simulink model "Robot_arm_position_control"  (Simulink 7.6)
settings: Solver=ode45  StartTime=0.0  StopTime=100  RelTol=1e-3
libraries: simulink x6, dspmtrx3 x1, powerlib x1
settings Model: Creator=Green  LastModifiedBy=Green

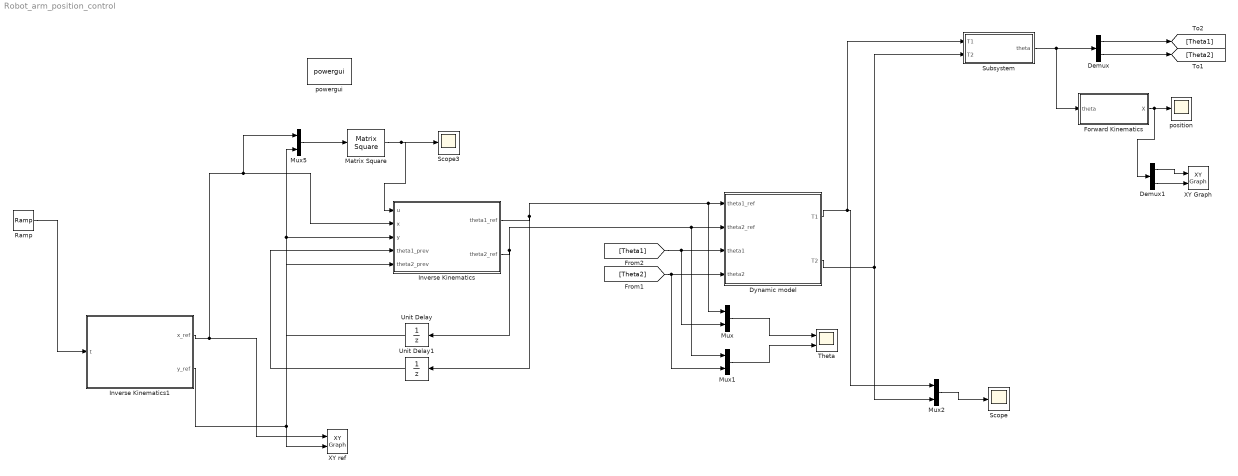
== system Robot_arm_position_control ==
  Demux : Demux  Outputs=2
  Demux1 : Demux  Outputs=2
  Dynamic model : Subsystem
  Forward Kinematics : Subsystem
  Inverse Kinematics : Stateflow chart  TreatAsAtomicUnit=on
  Inverse Kinematics1 : Stateflow chart  TreatAsAtomicUnit=on
  Matrix Square : dspmtrx3/Matrix Square  SystemSampleTime=-1  OutMin=[]  OutMax=[]
  Mux{,1..2,5} (4 alike) : Mux  Inputs=2
  Ramp : simulink/Sources/Ramp  SystemSampleTime=-1  slope=0.1  start=0  X0=0
  Scope : Scope
      settings: YMin=-1.1e+018  YMax=1.1e+018  SaveName=ScopeData2
  Scope3 : Scope
      settings: YMin=0.13  YMax=0.13  SaveName=ScopeData11
  Subsystem : Subsystem
  Theta : Scope  NumInputPorts=2
      settings: YMin=0.5~-1.2  YMax=1.45~0.7  SaveName=theta_graph  DataFormat=Structure
  Unit Delay : UnitDelay  SampleTime=-1
  Unit Delay1 : UnitDelay  SampleTime=-1
  XY Graph : simulink/Sinks/XY Graph  SystemSampleTime=-1  xmin=-0.5  xmax=0.5  ymin=-0.5  ymax=0.5  st=-1
  XY ref : simulink/Sinks/XY Graph  SystemSampleTime=-1  xmin=-0.5  xmax=0.5  ymin=-0.5  ymax=0.5  st=-1
  position : Scope
      settings: YMin=-0.05  YMax=0.4  SaveName=XY_graph  DataFormat=Array
  powergui : powerlib/powergui  Priority=1  SystemSampleTime=-1  SimulationMode=Discrete  SampleTime=50e-8  frequency=60  SPID=off  DisableSnubberDevices=off  DisableRonSwitches=off  DisableVfSwitches=off  SwTol=0  Interpol=off  frequencyindice=60  echomessages=off  HookPort=off  DisplayEquations=off  FunctionMessages=off  EnableUseOfTLC=off  x0status=blocks  RestoreLinks=warning  ResistiveCurrentMeasurement=off  Ylog=off  Xlog=on  ShowGrid=off  save=off  variable=ZData  ZoomFFT=off  StartTime=0.0  cycles=1  DisplayStyle=1  FreqAxis=off  MaxFrequency=1000  frequencyindicesteady=1  display=off  methode=off
  wires:
  Dynamic model/1(T1) -> Subsystem/1(T1), Mux2/1
  Dynamic model/2(T2) -> Subsystem/2(T2), Mux2/2
  [Theta2] -> Dynamic model/4(theta2), Mux1/2
  [Theta1] -> Dynamic model/3(theta1), Mux/2
  Inverse Kinematics/2(theta2_ref) -> Dynamic model/2(theta2_ref), Mux1/1, Unit Delay/1
  Mux/1 -> Theta/1
  Mux1/1 -> Theta/2
  Subsystem/1(theta) -> Demux/1, Forward Kinematics/1(theta)
  Demux/1 -> [Theta1]
  Demux/2 -> [Theta2]
  Mux2/1 -> Scope/1
  Inverse Kinematics/1(theta1_ref) -> Unit Delay1/1, Dynamic model/1(theta1_ref), Mux/1
  Unit Delay1/1 -> Inverse Kinematics/4(theta1_prev)
  Forward Kinematics/1(X) -> position/1, Demux1/1
  Demux1/1 -> XY Graph/1
  Demux1/2 -> XY Graph/2
  Mux5/1 -> Matrix Square/1
  Matrix Square/1 -> Scope3/1, Inverse Kinematics/1(u)
  Unit Delay/1 -> Inverse Kinematics/5(theta2_prev)
  Ramp/1 -> Inverse Kinematics1/1(t)
  Inverse Kinematics1/1(x_ref) -> XY ref/1, Inverse Kinematics/2(x), Mux5/1
  Inverse Kinematics1/2(y_ref) -> XY ref/2, Mux5/2, Inverse Kinematics/3(y)

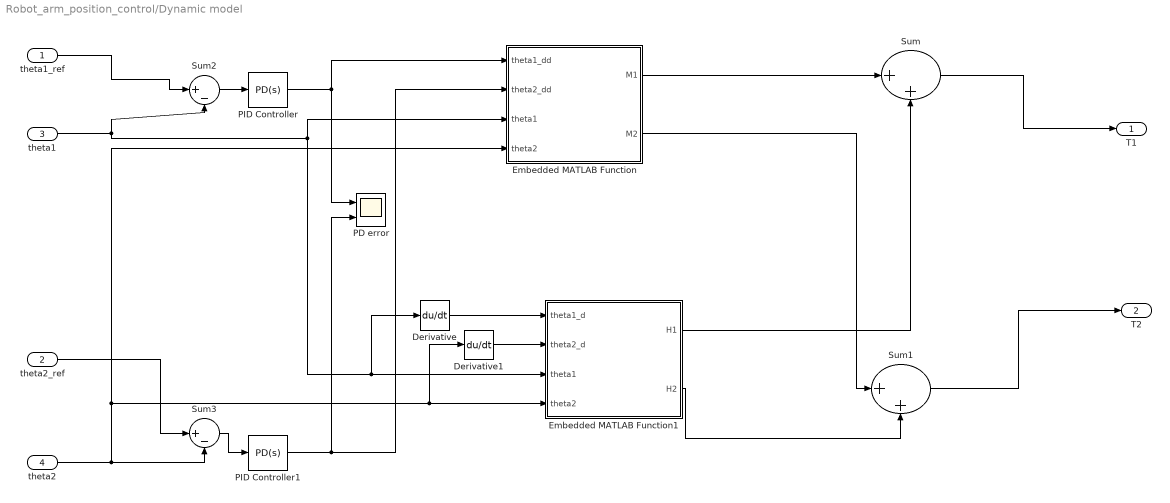
== system Robot_arm_position_control/Dynamic model ==
  theta1_ref : Inport
  theta2_ref : Inport  Port=2
  theta1 : Inport  Port=3
  theta2 : Inport  Port=4
  Derivative : Derivative
  Derivative1 : Derivative
  Embedded MATLAB Function : Stateflow chart  TreatAsAtomicUnit=on
  Embedded MATLAB Function1 : Stateflow chart  TreatAsAtomicUnit=on
  PD error : Scope  NumInputPorts=2
      settings: YMin=-3.25e+007~-4000  YMax=0~250  SaveName=ScopeData3
  PID Controller : simulink/Continuous/PID Controller  DialogController=pidpack.PIDConfig.pidDDGCreate  DialogControllerArgs=DataTag0  SystemSampleTime=-1  Controller=PD  TimeDomain=Continuous-time  SampleTime=1  IntegratorMethod=Forward Euler  FilterMethod=Forward Euler  Form=Ideal  P=220  I=1.92162729537983e-005  D=0.7  N=650  InitialConditionSource=internal  InitialConditionForIntegrator=0  InitialConditionForFilter=0  ExternalReset=none  LimitOutput=on  UpperSaturationLimit=1  LowerSaturationLimit=-1  LinearizeAsGain=off  AntiWindupMode=none  Kb=1  TrackingMode=off  Kt=1  PParamMin=[]  PParamMax=[]  IParamMin=[]  IParamMax=[]  DParamMin=[]  DParamMax=[]  NParamMin=[]  NParamMax=[]  KbParamMin=[]  KbParamMax=[]  KtParamMin=[]  KtParamMax=[]  POutMin=[]  POutMax=[]  IOutMin=[]  IOutMax=[]  DOutMin=[]  DOutMax=[]  NOutMin=[]  NOutMax=[]  KbOutMin=[]  KbOutMax=[]  KtOutMin=[]  KtOutMax=[]  IntegratorOutMin=[]  IntegratorOutMax=[]  FilterOutMin=[]  FilterOutMax=[]  SumOutMin=[]  SumOutMax=[]  SumI1OutMin=[]  SumI1OutMax=[]  SumI2OutMin=[]  SumI2OutMax=[]  SumI3OutMin=[]  SumI3OutMax=[]  SumDOutMin=[]  SumDOutMax=[]  SaturationOutMin=[]  SaturationOutMax=[]  IntegratorContinuousStateAttributes=''  IntegratorStateMustResolveToSignalObject=off  IntegratorRTWStateStorageClass=Auto  FilterContinuousStateAttributes=''  FilterStateMustResolveToSignalObject=off  FilterRTWStateStorageClass=Auto
  PID Controller1 : simulink/Continuous/PID Controller  DialogController=pidpack.PIDConfig.pidDDGCreate  DialogControllerArgs=DataTag1  SystemSampleTime=-1  Controller=PD  TimeDomain=Continuous-time  SampleTime=1  IntegratorMethod=Forward Euler  FilterMethod=Forward Euler  Form=Ideal  P=220  I=1  D=0.75  N=650  InitialConditionSource=internal  InitialConditionForIntegrator=0  InitialConditionForFilter=0  ExternalReset=none  LimitOutput=on  UpperSaturationLimit=1  LowerSaturationLimit=-1  LinearizeAsGain=off  AntiWindupMode=none  Kb=1  TrackingMode=off  Kt=1  PParamMin=[]  PParamMax=[]  IParamMin=[]  IParamMax=[]  DParamMin=[]  DParamMax=[]  NParamMin=[]  NParamMax=[]  KbParamMin=[]  KbParamMax=[]  KtParamMin=[]  KtParamMax=[]  POutMin=[]  POutMax=[]  IOutMin=[]  IOutMax=[]  DOutMin=[]  DOutMax=[]  NOutMin=[]  NOutMax=[]  KbOutMin=[]  KbOutMax=[]  KtOutMin=[]  KtOutMax=[]  IntegratorOutMin=[]  IntegratorOutMax=[]  FilterOutMin=[]  FilterOutMax=[]  SumOutMin=[]  SumOutMax=[]  SumI1OutMin=[]  SumI1OutMax=[]  SumI2OutMin=[]  SumI2OutMax=[]  SumI3OutMin=[]  SumI3OutMax=[]  SumDOutMin=[]  SumDOutMax=[]  SaturationOutMin=[]  SaturationOutMax=[]  IntegratorContinuousStateAttributes=''  IntegratorStateMustResolveToSignalObject=off  IntegratorRTWStateStorageClass=Auto  FilterContinuousStateAttributes=''  FilterStateMustResolveToSignalObject=off  FilterRTWStateStorageClass=Auto
  Sum : Sum  Inputs=|++
  Sum1 : Sum  Inputs=|++
  Sum2 : Sum  Inputs=|+-
  Sum3 : Sum  Inputs=|+-
  T1 : Outport
  T2 : Outport  Port=2
  wires:
  theta1_ref/1 -> Sum2/1
  theta1/1 -> Embedded MATLAB Function/3(theta1), Embedded MATLAB Function1/3(theta1), Derivative/1, Sum2/2
  theta2_ref/1 -> Sum3/1
  theta2/1 -> Embedded MATLAB Function/4(theta2), Embedded MATLAB Function1/4(theta2), Derivative1/1, Sum3/2
  Derivative/1 -> Embedded MATLAB Function1/1(theta1_d)
  Derivative1/1 -> Embedded MATLAB Function1/2(theta2_d)
  Embedded MATLAB Function/1(M1) -> Sum/1
  Embedded MATLAB Function1/1(H1) -> Sum/2
  Embedded MATLAB Function/2(M2) -> Sum1/1
  Embedded MATLAB Function1/2(H2) -> Sum1/2
  Sum/1 -> T1/1
  Sum1/1 -> T2/1
  PID Controller1/1 -> Embedded MATLAB Function/2(theta2_dd), PD error/2
  Sum2/1 -> PID Controller/1
  PID Controller/1 -> Embedded MATLAB Function/1(theta1_dd), PD error/1
  Sum3/1 -> PID Controller1/1

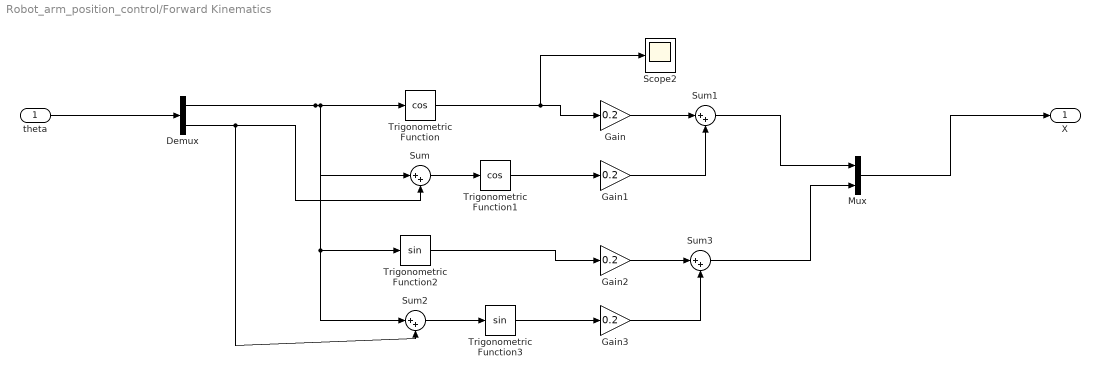
== system Robot_arm_position_control/Forward Kinematics ==
  theta : Inport
  Demux : Demux  Outputs=2
  Gain{,1..3} (4 alike) : Gain  Gain=0.2
  Mux : Mux  Inputs=2
  Scope2 : Scope
      settings: YMin=-1.1e+018  YMax=1.1e+018  SaveName=ScopeData10
  Sum{,1..3} (4 alike) : Sum  Inputs=|++
  Trigonometric Function : Trigonometry  Operator=cos
  Trigonometric Function1 : Trigonometry  Operator=cos
  Trigonometric Function2 : Trigonometry
  Trigonometric Function3 : Trigonometry
  X : Outport
  wires:
  theta/1 -> Demux/1
  Demux/1 -> Trigonometric Function/1, Sum/1, Sum2/1, Trigonometric Function2/1
  Demux/2 -> Sum/2, Sum2/2
  Sum/1 -> Trigonometric Function1/1
  Trigonometric Function/1 -> Gain/1, Scope2/1
  Trigonometric Function1/1 -> Gain1/1
  Sum1/1 -> Mux/1
  Sum2/1 -> Trigonometric Function3/1
  Trigonometric Function2/1 -> Gain2/1
  Trigonometric Function3/1 -> Gain3/1
  Sum3/1 -> Mux/2
  Gain/1 -> Sum1/1
  Gain1/1 -> Sum1/2
  Gain2/1 -> Sum3/1
  Gain3/1 -> Sum3/2
  Mux/1 -> X/1

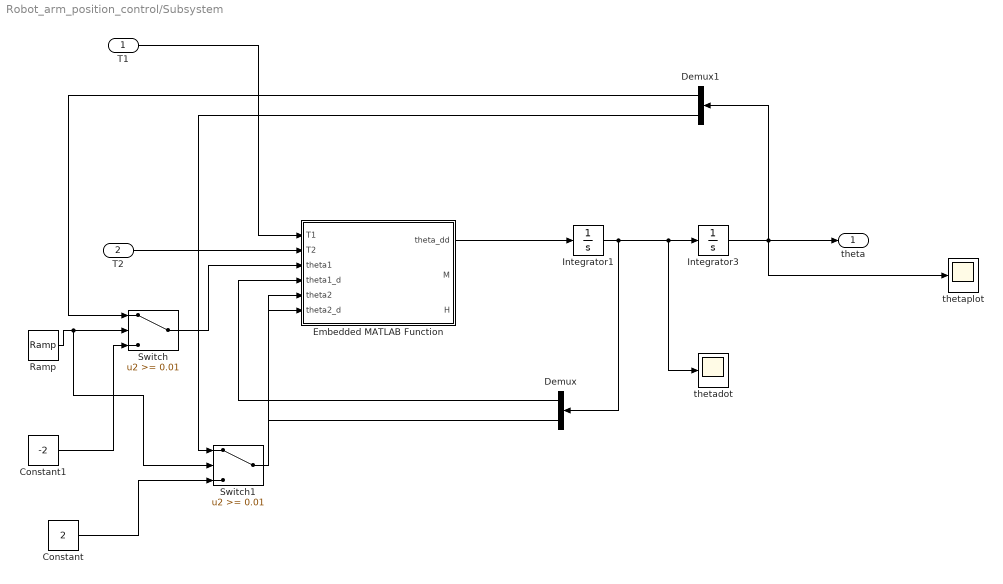
== system Robot_arm_position_control/Subsystem ==
  T1 : Inport
  T2 : Inport  Port=2
  Constant : Constant  Value=2
  Constant1 : Constant  Value=-2
  Demux : Demux  Outputs=2
  Demux1 : Demux  Outputs=2
  Embedded MATLAB Function : Stateflow chart  TreatAsAtomicUnit=on
  Integrator1 : Integrator  InitialCondition=30*pi/180
  Integrator3 : Integrator  InitialCondition=30*pi/180
  Ramp : simulink/Sources/Ramp  SystemSampleTime=-1  slope=1  start=0  X0=0
  Switch : Switch  Threshold=0.01
  Switch1 : Switch  Threshold=0.01
  thetadot : Scope
      settings: SaveName=ScopeData6
  thetaplot : Scope
      settings: YMin=0.5  YMax=12  SaveName=ScopeData5
  theta : Outport
  wires:
  T2/1 -> Embedded MATLAB Function/2(T2)
  T1/1 -> Embedded MATLAB Function/1(T1)
  Integrator1/1 -> Integrator3/1, thetadot/1, Demux/1
  Integrator3/1 -> theta/1, thetaplot/1, Demux1/1
  Embedded MATLAB Function/1(theta_dd) -> Integrator1/1
  Demux/1 -> Embedded MATLAB Function/4(theta1_d)
  Demux/2 -> Embedded MATLAB Function/6(theta2_d)
  Demux1/1 -> Switch/1
  Demux1/2 -> Switch1/1
  Ramp/1 -> Switch/2, Switch1/2
  Switch/1 -> Embedded MATLAB Function/3(theta1)
  Switch1/1 -> Embedded MATLAB Function/5(theta2)
  Constant1/1 -> Switch/3
  Constant/1 -> Switch1/3

== matlab function Dynamic model/Embedded MATLAB Function ==
  data: theta1_dd input double; M1 output double; theta2_dd input double; theta1 input double; theta2 input double; M2 output double
function [M1,M2] = fcn(theta1_dd,theta2_dd,theta1,theta2)
%#eml
% Leg parameters
m1 = 2; m2 = 2; l1 = 0.2; l2 = 0.2;
lc1 = l1/2; lc2 = l2/2; I1 = 0.02; I2 = 0.02;

% M(q)
m11 = m1*lc1^2+m2*(l1^2+lc2^2+2*l1*lc2*cos(theta2))+I1+I2;   
m12 = m2*(lc2^2+l1*lc2*cos(theta2))+I2;
m21 = m2*(lc2^2+l1*lc2*cos(theta2))+I2;
m22 = m2*lc2^2+I2;
M1 = m11*theta1_dd+m12*theta2_dd;
M2 = m21*theta1_dd+m22*theta2_dd;

== matlab function Dynamic model/Embedded MATLAB Function1 ==
  data: theta1_d input double; H1 output double; theta2_d input double; theta1 input double; theta2 input double; H2 output double
function [H1,H2] = fcn(theta1_d,theta2_d,theta1,theta2)
%#eml
% Leg parameters
m1 = 2; m2 = 2; l1 = 0.2; l2 = 0.2;
lc1 = l1/2; lc2 = l2/2; I1 = 0.02; I2 = 0.02;

% M(q)
H1 = (m1*lc2+m2*l1)*9.81*sin(theta1) + m2*lc2*9.81*sin(theta1+theta2) + (-m2*l1*lc2*theta2_d*sin(theta2))*theta1_d + (-m2*l1*lc2*(theta1_d + theta2_d)*sin(theta2))*theta2_d; 
H2 =  m2*lc2*9.81*sin(theta1 + theta2) + m2*l1*lc2*theta1_d*sin(theta2)*theta1_d;

== matlab function Inverse Kinematics1 ==
  data: t input double; x_ref output double; y_ref output double
function [x_ref,y_ref] = fcn(t)
%#eml

% Leg parameters
x_ref = 0.2 + 0.05*sin(3*t);
y_ref = 0.2 + 0.005*cos(3*t);

== matlab function Inverse Kinematics ==
  data: u input double; x input double; y input double; theta1_prev input double; theta2_prev input double; theta1_ref output double; theta2_ref output double
function [theta1_ref,theta2_ref] = fcn(u, x, y, theta1_prev, theta2_prev)
%#eml

% Leg parameters
l1 = 0.2; l2 = 0.2;
if u > 0.1599
    theta1_ref = theta1_prev;
    theta2_ref = theta2_prev;
    return
else
    C2 = (x^2+y^2-l1^2-l2^2)/(2*l1*l2);
    if -1>C2>1
        theta1_ref = theta1_prev;
        theta2_ref = theta2_prev;
        C1 = 0;
        return
    end
    S2 = sqrt(1-C2^2);
    theta2_ref = atan2(-S2,C2);

    C1 = ((l1+l2*C2)*x - (l2*S2*y))/(x^2+y^2);
    if -1>C1>1
        theta1_ref = theta1_prev;
        theta2_ref = theta2_prev;
        return
    end
    % S1 = ((l1+l2)*y + (l2*S2*x))/(x^2+y^2);
    S1 = sqrt(1-C1^2);
    theta1_ref = atan2(S1,C1);
end

% X = [x; y];


% J = [-l1*sin(theta1)-l2*sin(theta1 + theta2) -l2*sin(theta1 + theta2); l1*cos(theta1)+l2*cos(theta1 + theta2) l2*cos(theta1 + theta2)];
% InvJ = inv(J);
% 
% theta_ref = InvJ*X;
% theta1_ref = theta_ref(1);
% theta2_ref = theta_ref(2);

== matlab function Subsystem/Embedded MATLAB Function ==
  data: theta_dd output double; T1 input double; T2 input double; theta1 input double; theta1_d input double; M output double; H output double; theta2 input double; theta2_d input double
function [theta_dd, M, H] = fcn(T1,T2,theta1,theta1_d,theta2,theta2_d)
%#eml
% Leg parameters
m1 = 2; m2 = 2; l1 = 0.2; l2 = 0.2;
lc1 = l1/2; lc2 = l2/2; I1 = 0.02; I2 = 0.02;
T = [T1; T2];

% M(q)
m11 = m1*lc1^2+m2*(l1^2+lc2^2+2*l1*lc2*cos(theta2))+I1+I2;   
m12 = m2*(lc2^2+l1*lc2*cos(theta2))+I2;
m21 = m2*(lc2^2+l1*lc2*cos(theta2))+I2;
m22 = m2*lc2^2+I2;
M = [m11,m12;m21,m22];

% H(q)
H1 = (m1*lc2+m2*l1)*9.81*sin(theta1) + m2*lc2*9.81*sin(theta1+theta2) + (-m2*l1*lc2*theta2_d*sin(theta2))*theta1_d + (-m2*l1*lc2*(theta1_d + theta2_d)*sin(theta2))*theta2_d; 
H2 =  m2*lc2*9.81*sin(theta1 + theta2) + m2*l1*lc2*theta1_d*sin(theta2)*theta1_d;
H = [H1; H2];

% Inverse M(q)
% InvM = inv(M);
% Im11 = InvM(1,1); Im12 = InvM(1,2);
% Im21 = InvM(2,1); Im22 = InvM(2,2);

% theta1_dd = (Im11*(T1-H1)+Im12*(T2-H2));
% theta2_dd = (Im21*(T1-H1)+Im22*(T2-H2));
% theta_dd = [theta1_dd; theta2_dd]; 

theta_dd = inv(M)*(T-H);
